simulink model "TF_RLCsimulink"  (R2025b)
settings: Solver=VariableStepAuto  StartTime=0.0  StopTime=0.25e-3  RelTol=1e-3
libraries: fl_lib x25, nesl_utility x12
settings Model: Creator=Brayan Barragan  LastModifiedBy=Brayan Barragan

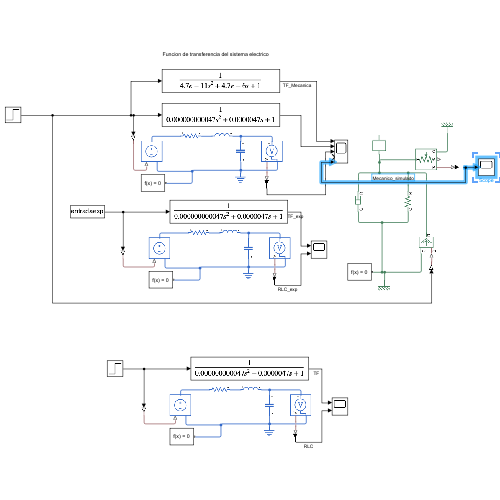
[thumbnail: Simulink's stored preview of the top-level diagram]
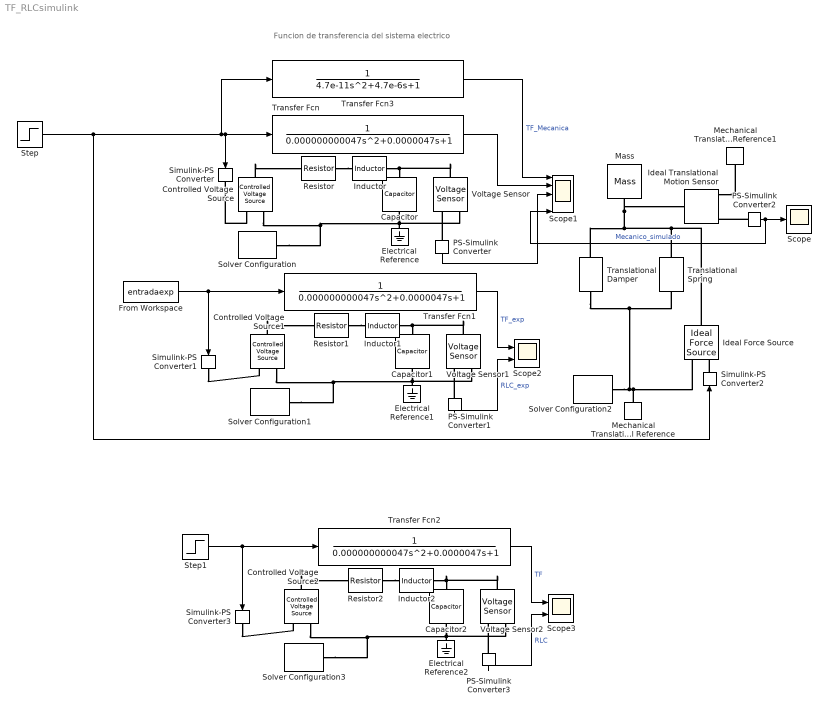
== system TF_RLCsimulink ==
  note: Funcion de transferencia del sistema electrico
  Capacitor : fl_lib/Electrical/Electrical Elements/Capacitor  c=10e-9 F  r=1e-6 Ohm  g=0 1/Ohm  i_specify=off  i_priority=None  i=0 A  i_nominal_specify=off  i_nominal_value=1  i_nominal_unit=A  v_specify=off  v_priority=None  v=0 V  v_nominal_specify=off  v_nominal_value=1  v_nominal_unit=V  vc_specify=off  vc_priority=High  vc=0 V  vc_nominal_specify=off  vc_nominal_value=1  vc_nominal_unit=V
  Capacitor1 : fl_lib/Electrical/Electrical Elements/Capacitor  c=10e-9 F  r=1e-6 Ohm  g=0 1/Ohm  i_specify=off  i_priority=None  i=0 A  i_nominal_specify=off  i_nominal_value=1  i_nominal_unit=A  v_specify=off  v_priority=None  v=0 V  v_nominal_specify=off  v_nominal_value=1  v_nominal_unit=V  vc_specify=off  vc_priority=High  vc=0 V  vc_nominal_specify=off  vc_nominal_value=1  vc_nominal_unit=V
  Capacitor2 : fl_lib/Electrical/Electrical Elements/Capacitor  c=10e-9 F  r=1e-6 Ohm  g=0 1/Ohm  i_specify=off  i_priority=None  i=0 A  i_nominal_specify=off  i_nominal_value=1  i_nominal_unit=A  v_specify=off  v_priority=None  v=0 V  v_nominal_specify=off  v_nominal_value=1  v_nominal_unit=V  vc_specify=off  vc_priority=High  vc=0 V  vc_nominal_specify=off  vc_nominal_value=1  vc_nominal_unit=V
  Controlled Voltage Source : fl_lib/Electrical/Electrical Sources/Controlled Voltage Source
  Controlled Voltage Source1 : fl_lib/Electrical/Electrical Sources/Controlled Voltage Source
  Controlled Voltage Source2 : fl_lib/Electrical/Electrical Sources/Controlled Voltage Source
  Electrical Reference : fl_lib/Electrical/Electrical Elements/Electrical Reference
  Electrical Reference1 : fl_lib/Electrical/Electrical Elements/Electrical Reference
  Electrical Reference2 : fl_lib/Electrical/Electrical Elements/Electrical Reference
  From Workspace : FromWorkspace  VariableName=entradaexp  SampleTime=-1  OutputAfterFinalValue=Setting to zero
  Ideal Force Source : fl_lib/Mechanical/Mechanical Sources/Ideal Force Source
  Ideal Translational Motion Sensor : fl_lib/Mechanical/Mechanical Sensors/Ideal Translational Motion Sensor  reference=foundation.enum.MeasurementReference.difference  acceleration_port=false  velocity_port=true  position_port=true  offset=0 m
  Inductor : fl_lib/Electrical/Electrical Elements/Inductor  l=4.7e-3 H  r=0 Ohm  g=1e-9 1/Ohm  i_specify=off  i_priority=None  i=0 A  i_nominal_specify=off  i_nominal_value=1  i_nominal_unit=A  v_specify=off  v_priority=None  v=0 V  v_nominal_specify=off  v_nominal_value=1  v_nominal_unit=V  i_L_specify=off  i_L_priority=High  i_L=0 A  i_L_nominal_specify=off  i_L_nominal_value=1  i_L_nominal_unit=A
  Inductor1 : fl_lib/Electrical/Electrical Elements/Inductor  l=4.7e-3 H  r=0 Ohm  g=1e-9 1/Ohm  i_specify=off  i_priority=None  i=0 A  i_nominal_specify=off  i_nominal_value=1  i_nominal_unit=A  v_specify=off  v_priority=None  v=0 V  v_nominal_specify=off  v_nominal_value=1  v_nominal_unit=V  i_L_specify=off  i_L_priority=High  i_L=0 A  i_L_nominal_specify=off  i_L_nominal_value=1  i_L_nominal_unit=A
  Inductor2 : fl_lib/Electrical/Electrical Elements/Inductor  l=4.7e-3 H  r=0 Ohm  g=1e-9 1/Ohm  i_specify=off  i_priority=None  i=0 A  i_nominal_specify=off  i_nominal_value=1  i_nominal_unit=A  v_specify=off  v_priority=None  v=0 V  v_nominal_specify=off  v_nominal_value=1  v_nominal_unit=V  i_L_specify=off  i_L_priority=High  i_L=0 A  i_L_nominal_specify=off  i_L_nominal_value=1  i_L_nominal_unit=A
  Mass : fl_lib/Mechanical/Translational Elements/Mass  mass=4.7e-11 kg  num_ports=foundation.enum.numPorts2.one  v_specify=off  v_priority=High  v=0 m/s  v_nominal_specify=off  v_nominal_value=1  v_nominal_unit=m/s  f_specify=off  f_priority=None  f=0 N  f_nominal_specify=off  f_nominal_value=1  f_nominal_unit=N
  Mechanical Translational Reference : fl_lib/Mechanical/Translational Elements/Mechanical Translational Reference
  Mechanical Translational Reference1 : fl_lib/Mechanical/Translational Elements/Mechanical Translational Reference
  PS-Simulink Converter{,1..3} (4 alike) : nesl_utility/PS-Simulink Converter  PhysicalDomain=network_engine_domain  SubClassName=ps_output  LeftPortType=input  RightPortType=output  PseudoPeriodic=off  Frequencies=[]  VectorFormat=inherit  Unit=inherit  AffineConversion=off
  Resistor : fl_lib/Electrical/Electrical Elements/Resistor  R=470 Ohm  i_specify=off  i_priority=None  i=0 A  i_nominal_specify=off  i_nominal_value=1  i_nominal_unit=A  v_specify=off  v_priority=None  v=0 V  v_nominal_specify=off  v_nominal_value=1  v_nominal_unit=V
  Resistor1 : fl_lib/Electrical/Electrical Elements/Resistor  R=470 Ohm  i_specify=off  i_priority=None  i=0 A  i_nominal_specify=off  i_nominal_value=1  i_nominal_unit=A  v_specify=off  v_priority=None  v=0 V  v_nominal_specify=off  v_nominal_value=1  v_nominal_unit=V
  Resistor2 : fl_lib/Electrical/Electrical Elements/Resistor  R=470 Ohm  i_specify=off  i_priority=None  i=0 A  i_nominal_specify=off  i_nominal_value=1  i_nominal_unit=A  v_specify=off  v_priority=None  v=0 V  v_nominal_specify=off  v_nominal_value=1  v_nominal_unit=V
  Scope : Scope
      settings: ActiveDisplayYMinimum=-0.16472266700556176  ActiveDisplayYMaximum=1.482504003050056  DataLoggingVariableName=ScopeData2
  Scope1 : Scope  NumInputPorts=5
      settings: SampleTime=0.25e-3/1000  ActiveDisplayYMinimum=-0.16472266700556176  ActiveDisplayYMaximum=1.482504003050056
  Scope2 : Scope  NumInputPorts=2
      settings: SampleTime=0.25e-3/1000  ActiveDisplayYMinimum=-1.9996231426498212  ActiveDisplayYMaximum=1.9746580004525665
  Scope3 : Scope  NumInputPorts=2
      settings: SampleTime=0.25e-3/1000  ActiveDisplayYMinimum=-0.16472266700556176  ActiveDisplayYMaximum=1.482504003050056  DataLoggingVariableName=ScopeData3
  Simulink-PS Converter{,1..3} (4 alike) : nesl_utility/Simulink-PS Converter  PhysicalDomain=network_engine_domain  SubClassName=ps_input  LeftPortType=input  RightPortType=output  PseudoPeriodic=off  Frequencies=[]  NoiseDistribution=none  NoiseParameters=[]  Unit=1  AffineConversion=off  FilteringAndDerivatives=provide  SimscapeFilterOrder=1  InputFilterTimeConstant=0.001  UdotUserProvided=0
  Solver Configuration{,1..3} (4 alike) : nesl_utility/Solver Configuration  PhysicalDomain=network_engine_domain  SubClassName=solver  LeftPortType=input  RightPortType=generic  Tones=[]  Harmonics=[]  SimulateNoise=off  Profile=off  UseLocalSampling=off  EnableSwitchedLinearOptims=on  FrequencyDomain=off  UseCCode=off  RelTol=0.001  AbsTol=0.001  MinStep=1e-09  ToWorkspace=off  RevertToSquareIcSolve=off  NumHomotopyIterations=100  PhasorMode=off  PhasorModeNumHarmonics=1  ConsistencySolver=NEWTON_XTOL_AFTER_FTOL  IndexReductionMethod=DerivativeReplacement  DoDC=off  ResidualTolerance=1e-09  ConsistencyTolSource=GLOBAL  ConsistencyAbsTol=0.001  ConsistencyRelTol=0.001  ConsistencyTolFactor=0.001  UseLocalSolver=off  LocalSolverChoice=NE_BACKWARD_EULER_ADVANCER  ResolveIndetEquations=on  FunctionEvalNumThread=1  LocalSolverSampleTime=0.001  DoFixedCost=off  MaxNonlinIter=3  MaxModeIter=2  ComputeImpulses=off  ImpulseIterations=2  LinearAlgebra=auto  LinearAlgebraNumThread=0  EquationFormulation=NE_TIME_EF  DelaysMemoryBudget=1024  AutomaticFiltering=on  FilteringTimeConstant=0.001  PartitionStorageMethod=AS_NEEDED  PartitionMemoryBudget=1024  PartitionMethod=ROBUST  MultibodyUseLocalSolver=off  MultibodyLocalSolverChoice=ODE1  MultibodyLocalSolverSampleTime=0.001
  Step : Step  Time=0  SampleTime=0
  Step1 : Step  Time=0  SampleTime=0
  Transfer Fcn : TransferFcn  Denominator=[0.000000000047 0.0000047 1]
  Transfer Fcn1 : TransferFcn  Denominator=[0.000000000047 0.0000047 1]
  Transfer Fcn2 : TransferFcn  Denominator=[0.000000000047 0.0000047 1]
  Transfer Fcn3 : TransferFcn  Denominator=[4.7e-11 4.7e-6 1]
  Translational Damper : fl_lib/Mechanical/Translational Elements/Translational Damper  D=4.7e-6 N*s/m  v_specify=off  v_priority=None  v=0 m/s  v_nominal_specify=off  v_nominal_value=1  v_nominal_unit=m/s  f_specify=off  f_priority=None  f=0 N  f_nominal_specify=off  f_nominal_value=1  f_nominal_unit=N
  Translational Spring : fl_lib/Mechanical/Translational Elements/Translational Spring  spr_rate=1 N/m  v_specify=off  v_priority=None  v=0 m/s  v_nominal_specify=off  v_nominal_value=1  v_nominal_unit=m/s  f_specify=off  f_priority=None  f=0 N  f_nominal_specify=off  f_nominal_value=1  f_nominal_unit=N  x_specify=off  x_priority=High  x=0 m  x_nominal_specify=off  x_nominal_value=1  x_nominal_unit=m
  Voltage Sensor : fl_lib/Electrical/Electrical Sensors/Voltage Sensor
  Voltage Sensor1 : fl_lib/Electrical/Electrical Sensors/Voltage Sensor
  Voltage Sensor2 : fl_lib/Electrical/Electrical Sensors/Voltage Sensor
  wires:
  Step/1 -> Simulink-PS Converter2/1, Transfer Fcn3/1, Simulink-PS Converter/1, Transfer Fcn/1
  Transfer Fcn/1 -> Scope1/2
  PS-Simulink Converter/1 -> Scope1/3
  Transfer Fcn1/1 -> Scope2/1  "TF_exp"
  PS-Simulink Converter1/1 -> Scope2/2  "RLC_exp"
  From Workspace/1 -> Simulink-PS Converter1/1, Transfer Fcn1/1
  Transfer Fcn3/1 -> Scope1/1  "TF_Mecanica"
  PS-Simulink Converter2/1 -> Scope1/5, Scope/1  "Mecanico_simulado"
  Step1/1 -> Simulink-PS Converter3/1, Transfer Fcn2/1
  Transfer Fcn2/1 -> Scope3/1  "TF"
  PS-Simulink Converter3/1 -> Scope3/2  "RLC"
  connections:
  Capacitor/RConn1 -- Controlled Voltage Source/RConn2 -- Solver Configuration/RConn1 -- Voltage Sensor/RConn2 -- Electrical Reference/LConn1
  Voltage Sensor/LConn1 -- Inductor/RConn1 -- Capacitor/LConn1
  PS-Simulink Converter/LConn1 -- Voltage Sensor/RConn1
  Controlled Voltage Source/RConn1 -- Simulink-PS Converter/RConn1
  Resistor/RConn1 -- Inductor/LConn1
  Controlled Voltage Source/LConn1 -- Resistor/LConn1
  Electrical Reference1/LConn1 -- Capacitor1/RConn1 -- Controlled Voltage Source1/RConn2 -- Solver Configuration1/RConn1 -- Voltage Sensor1/RConn2
  Inductor1/RConn1 -- Voltage Sensor1/LConn1 -- Capacitor1/LConn1
  PS-Simulink Converter1/LConn1 -- Voltage Sensor1/RConn1
  Simulink-PS Converter1/RConn1 -- Controlled Voltage Source1/RConn1
  Resistor1/RConn1 -- Inductor1/LConn1
  Controlled Voltage Source1/LConn1 -- Resistor1/LConn1
  Translational Spring/LConn1 -- Translational Damper/LConn1 -- Ideal Translational Motion Sensor/LConn1 -- Mass/LConn1 -- Ideal Force Source/LConn1
  Mechanical Translational Reference/LConn1 -- Translational Spring/RConn1 -- Translational Damper/RConn1 -- Solver Configuration2/RConn1 -- Ideal Force Source/RConn2
  PS-Simulink Converter2/LConn1 -- Ideal Translational Motion Sensor/RConn3
  Ideal Translational Motion Sensor/RConn1 -- Mechanical Translational Reference1/LConn1
  Simulink-PS Converter2/RConn1 -- Ideal Force Source/RConn1
  Solver Configuration3/RConn1 -- Electrical Reference2/LConn1 -- Capacitor2/RConn1 -- Voltage Sensor2/RConn2 -- Controlled Voltage Source2/RConn2
  Capacitor2/LConn1 -- Inductor2/RConn1 -- Voltage Sensor2/LConn1
  PS-Simulink Converter3/LConn1 -- Voltage Sensor2/RConn1
  Simulink-PS Converter3/RConn1 -- Controlled Voltage Source2/RConn1
  Controlled Voltage Source2/LConn1 -- Resistor2/LConn1
  Resistor2/RConn1 -- Inductor2/LConn1
